simulink model "acceleration"  (R2019a)
settings: Solver=ode45  StartTime=0.0  StopTime=10  MaxStep=0.0001  RelTol=1e-3
settings Model: Creator=ChairmanYang1966  LastModifiedBy=ChairmanYang1966

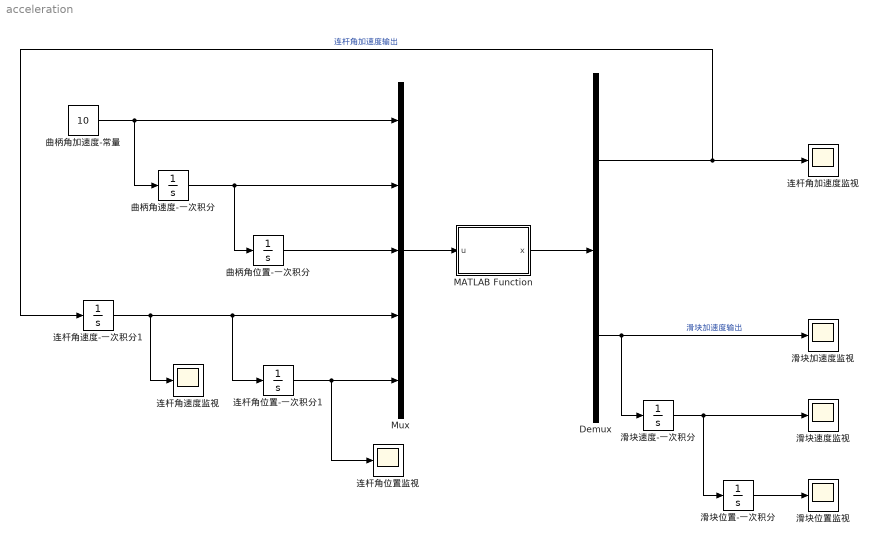
== system acceleration ==
  Demux : Demux  Outputs=2
  MATLAB Function : MATLAB Function  TreatAsAtomicUnit=on
  Mux : Mux  Inputs=5
  曲柄角位置-一次积分 : Integrator
  曲柄角加速度-常量 : Constant  Value=10
  曲柄角速度-一次积分 : Integrator
  滑块位置-一次积分 : Integrator  InitialCondition=70
  滑块位置监视 : Scope
  滑块加速度监视 : Scope
  滑块速度-一次积分 : Integrator
  滑块速度监视 : Scope
  连杆角位置-一次积分1 : Integrator
  连杆角位置监视 : Scope
  连杆角加速度监视 : Scope
  连杆角速度-一次积分1 : Integrator
  连杆角速度监视 : Scope
  wires:
  Mux/1 -> MATLAB Function/1(u)
  MATLAB Function/1(x) -> Demux/1
  Demux/2 -> 滑块加速度监视/1, 滑块速度-一次积分/1  "滑块加速度输出"
  滑块速度-一次积分/1 -> 滑块速度监视/1, 滑块位置-一次积分/1
  滑块位置-一次积分/1 -> 滑块位置监视/1
  Demux/1 -> 连杆角速度-一次积分1/1, 连杆角加速度监视/1  "连杆角加速度输出"
  曲柄角加速度-常量/1 -> 曲柄角速度-一次积分/1, Mux/1
  曲柄角位置-一次积分/1 -> Mux/3
  曲柄角速度-一次积分/1 -> 曲柄角位置-一次积分/1, Mux/2
  连杆角位置-一次积分1/1 -> 连杆角位置监视/1, Mux/5
  连杆角速度-一次积分1/1 -> 连杆角速度监视/1, Mux/4, 连杆角位置-一次积分1/1

== matlab function acceleration/MATLAB Function ==
  data: u input; x output
function x = compa(u)
r1=15;r2=55;
a=[r2*sin(u(5)) 1;r2*cos(u(5)) 0];
b=[-r1*cos(u(3))*u(2)^2-r2*cos(u(5))*u(4)^2-r1*sin(u(3))*u(1);r1*sin(u(3))*u(2)^2+r2*sin(u(5))*u(4)^2-r1*cos(u(3))*u(1)];
x = inv(a)*b;
%曲柄长15mm，连杆长55mm
%u(1)指征曲柄角加速度，u(2)指征曲柄角速度，u(3)指征曲柄角位置，u(4)指征连杆角速度，u(5)指示连杆角位置
%x(1)指征连杆角加速度，x(2)指征滑块加速度
